simulink model "Model_3_Hieu_1_12"  (R2021a)
settings: Solver=VariableStepAuto  StartTime=0.0  StopTime=10  RelTol=1e-3
InitFcn:
  | ml=0.2;
  | mc=0.5;
  | mt=0.5;
  | g=9.81;
  | l_ref=0.5;
  | l_ini=0.5;
  | l=l_ini;
  | n1=5;n2=1;
  | x_ref=10;
  | 
  | %ADRC' s parameter caculation
  | %b0 = (ml+mc)/(mc*ml +mc*mt+ml*mt); %Hieu
  | b0=(ml+mc)/(mt*mc+2*ml*mc+mt*ml+ml^2+mc^2); %Enhanced-coupling
  | k_ESO = 50;
  | T_set  = 6;
  | 
  | s_cl = -5.85/T_set;
  | Kp   = s_cl^2;
  | Kd   = -2*s_cl;
  | 
  | s_ESO = k_ESO*s_cl;
  | l1        = -3*s_ESO;
  | l2        = 3*( s_ESO)^2;
  | l3        = -(s_ESO)^3;
  | 
  | %Observer
  | A = [-l1, 1, 0;
  |         -l2, 0, 1;
  |         -l3, 0, 0];
  | B = [0;
  |         b0;
  |         0];
  | L = [l1;
  |        l2;
  |        l3];
  | 
  | %b1 = (mt+mc)/(mc*ml +mc*mt+ml*mt);
  | b1=1/(ml+mc);
  | k_ESO1 =100;
  | T_set1  = 3;
  | s_cl1 = -5.85/T_set1;
  | Kp1   = s_cl1^2;
  | Kd1   = -2*s_cl1;
  | 
  | s_ESO1 = k_ESO1*s_cl1;
  | l11        = -3*s_ESO1;
  | l21        = 3*( s_ESO1)^2;
  | l31        = -(s_ESO1)^3;
  | 
  | %Observer
  | A1 = [-l11, 1, 0;
  |         -l21, 0, 1;
  |         -l31, 0, 0];
  | B1 = [0;
  |         b1;
  |         0];
  | L1 = [l11;
  |        l21;
  |        l31];
  | 
  | L1=l_ini;
  | L2=0.2;
  | m1=0.2;
  | m2=0.5;
  | m=0.5;
  | %Bo input shaping
  | alpha = (1/L1 + 1/L2)*(m1+m2)/m1;
  | beta = (((m1+m2)/m1)^2)*((1/L1 + 1/L2)^2) - 4*(m1+m2)/(m1*L1*L2);
  | w1 = sqrt(g*(alpha - sqrt(beta))/2);
  | w2 = sqrt(g*(alpha + sqrt(beta))/2);
  | damping_ratio = 0;
  | wd1 = w1*sqrt(1-damping_ratio^2);
  | wd2 = w2*sqrt(1-damping_ratio^2);
  | k = exp(damping_ratio*pi/sqrt(1-damping_ratio^2));
  | 
  | %ETM4_1
  | m_etm4_1 = 0.1;
  | I_etm4_1 = (1+m_etm4_1)*k*k/(k^2 + (1+m_etm4_1)*(k^(4/3)+k^(2/3)) + m_etm4_1);
  | A1_etm4_1 = I_etm4_1/(1+m_etm4_1);
  | A2_etm4_1 = I_etm4_1/(k^(2/3));
  | A3_etm4_1 = I_etm4_1/(k^(4/3));
  | A4_etm4_1 = m_etm4_1*I_etm4_1/((1+m_etm4_1)*(k^2));
  | t1_etm4_1 = (2*pi/3)/wd1;
  | t2_etm4_1 = (4*pi/3)/wd1;
  | t3_etm4_1 = 2*pi/wd1;
  | %ETM4_2
  | m_etm4_2 = 0.1;
  | I_etm4_2 = (1+m_etm4_2)*k*k/(k^2 + (1+m_etm4_2)*(k^(4/3)+k^(2/3)) + m_etm4_2);
  | A1_etm4_2 = I_etm4_2/(1+m_etm4_2);
  | A2_etm4_2 = I_etm4_2/(k^(2/3));
  | A3_etm4_2 = I_etm4_2/(k^(4/3));
  | A4_etm4_2 = m_etm4_2*I_etm4_2/((1+m_etm4_2)*(k^2));
  | t1_etm4_2 = (2*pi/3)/wd2;
  | t2_etm4_2 = (4*pi/3)/wd2;
  | t3_etm4_2 = 2*pi/wd2;
values from neighbouring files (symbols this model uses):
  particle = repmat(empty_particle, nPop, 1)    [PSO16_12.m]    (also in PSO_ZVD.m)
undefined symbols (not defined in the file or in its folder): i
libraries: neural x35, simulink_extras x11, simulink x5
(part 1 of 15)
settings Model: Creator=Dao Hieu  LastModifiedBy=Admin

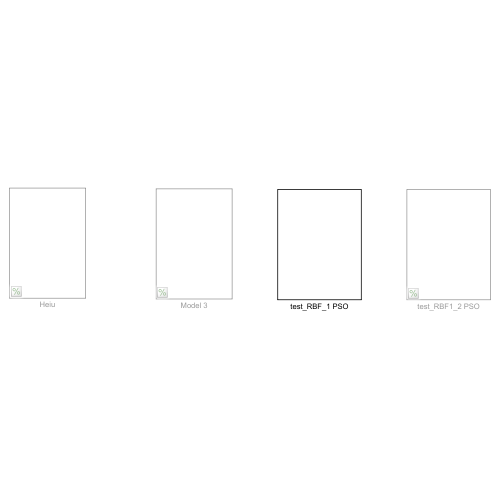
[thumbnail: Simulink's stored preview of the top-level diagram]
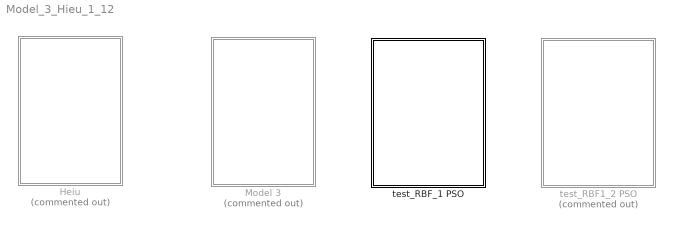
== system Model_3_Hieu_1_12 ==
  Heiu : Subsystem  Commented=on
  Model 3 : Subsystem  Commented=on
  test_RBF1_2 PSO : Subsystem  Commented=on
  test_RBF_1 PSO : Subsystem

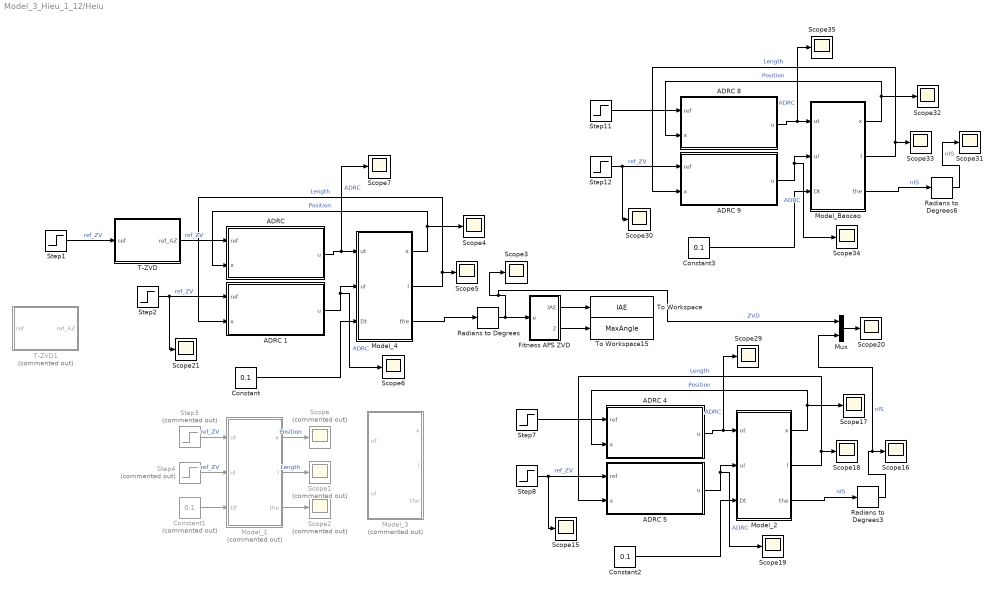
== system Model_3_Hieu_1_12/Heiu ==
  "ADRC " : Subsystem
  ADRC 1 : Subsystem
  ADRC 4 : Subsystem
  ADRC 5 : Subsystem
  ADRC 8 : Subsystem
  ADRC 9 : Subsystem
  Constant : Constant  Value=0.1
  Constant1 : Constant  Commented=on  Value=0.1
  Constant2 : Constant  Value=0.1
  Constant3 : Constant  Value=0.1
  Fitness APS ZVD : Subsystem
  Model_1 : Subsystem  Commented=on
  Model_2 : Subsystem
  Model_3 : Subsystem  Commented=on
  Model_4 : Subsystem
  Model_Baocao : Subsystem
  Mux : Mux  Inputs=2
  Radians to Degrees : simulink_extras/Transformations/Radians to Degrees
  Radians to Degrees3 : simulink_extras/Transformations/Radians to Degrees
  Radians to Degrees6 : simulink_extras/Transformations/Radians to Degrees
  Scope : Scope  Commented=on
  Scope1 : Scope  Commented=on
  Scope{3..7,15..21,29..35} (19 alike) : Scope
  Scope2 : Scope  Commented=on
  Step1 : Step  SampleTime=0
  Step11 : Step  SampleTime=0
  Step12 : Step  Before=l_ini  After=l_ref  SampleTime=0
  Step2 : Step  Before=l_ini  After=l_ref  SampleTime=0
  Step3 : Step  Commented=on  SampleTime=0
  Step4 : Step  Commented=on  Before=l  After=l  SampleTime=0
  Step7 : Step  SampleTime=0
  Step8 : Step  Before=l_ini  After=l_ref  SampleTime=0
  T-ZVD : Subsystem
  T-ZVD1 : Subsystem  Commented=on
  To Workspace : ToWorkspace  VariableName=IAE  SampleTime=-1
  To Workspace15 : ToWorkspace  VariableName=MaxAngle  SampleTime=-1
  wires:
  Model_4/1(x) -> Scope4/1, "ADRC "/2(x)  "Position"
  Model_4/3(the) -> Radians to Degrees/1
  Step12/1 -> Scope30/1, ADRC 9/1(ref)  "ref_ZV"
  "ADRC "/1(u) -> Scope7/1, Model_4/1(ut)  "ADRC"
  Model_Baocao/2(l) -> Scope33/1, ADRC 9/2(x)  "Length"
  Mux/1 -> Scope20/1
  Radians to Degrees6/1 -> Scope31/1  "nIS"
  Model_2/1(x) -> ADRC 4/2(x), Scope17/1  "Position"
  Fitness APS ZVD/1(IAE) -> To Workspace/1
  Step8/1 -> ADRC 5/1(ref), Scope15/1  "ref_ZV"
  Fitness APS ZVD/2(MAx) -> To Workspace15/1
  ADRC 1/1(u) -> Scope6/1, Model_4/2(ul)  "ADRC"
  Step11/1 -> ADRC 8/1(ref)
  Radians to Degrees/1 -> Mux/1, Scope3/1, Fitness APS ZVD/1(e)  "ZVD"
  Constant3/1 -> Model_Baocao/3(Dt)
  Step4/1 -> Model_1/2(ul)  "ref_ZV"
  Step2/1 -> Scope21/1, ADRC 1/1(ref)  "ref_ZV"
  Model_1/1(x) -> Scope/1  "Position"
  ADRC 5/1(u) -> Scope19/1, Model_2/2(ul)  "ADRC"
  Model_2/3(the) -> Radians to Degrees3/1  "nIS"
  Model_1/3(the) -> Scope2/1
  ADRC 8/1(u) -> Scope35/1, Model_Baocao/1(ut)  "ADRC"
  Constant/1 -> Model_4/3(Dt)
  Step1/1 -> T-ZVD/1(ref)  "ref_ZV"
  Step3/1 -> Model_1/1(ut)  "ref_ZV"
  ADRC 4/1(u) -> Scope29/1, Model_2/1(ut)  "ADRC"
  Radians to Degrees3/1 -> Mux/2, Scope16/1  "nIS"
  T-ZVD/1(ref_AZ) -> "ADRC "/1(ref)  "ref_ZV"
  Model_2/2(l) -> ADRC 5/2(x), Scope18/1  "Length"
  ADRC 9/1(u) -> Scope34/1, Model_Baocao/2(ul)  "ADRC"
  Constant2/1 -> Model_2/3(Dt)
  Model_Baocao/1(x) -> Scope32/1, ADRC 8/2(x)  "Position"
  Model_Baocao/3(the) -> Radians to Degrees6/1  "nIS"
  Constant1/1 -> Model_1/3(Dt)
  Step7/1 -> ADRC 4/1(ref)
  Model_1/2(l) -> Scope1/1  "Length"
  Model_4/2(l) -> Scope5/1, ADRC 1/2(x)  "Length"

== system Model_3_Hieu_1_12/Model 3 ==
  ADRC 10 : Subsystem
  ADRC 11 : Subsystem
  ADRC 6 : Subsystem
  ADRC 7 : Subsystem
  ETM2 : Subsystem
  Mux1 : Mux  Inputs=2
  Mux2 : Mux  Inputs=2
  Radians to Degrees{4..5,7..8} (4 alike) : simulink_extras/Transformations/Radians to Degrees
  Scope{22..28,36..43} (15 alike) : Scope
  Step10 : Step  Before=l_ini  After=l_ref  SampleTime=0
  Step13 : Step  Before=l_ini  After=l_ref  SampleTime=0
  Step14 : Step  SampleTime=0
  Step9 : Step  SampleTime=0
  Theta1 : Scope
  Theta2 : Scope
  enhanced : Subsystem
  enhanced1 : Subsystem
  wires:
  Radians to Degrees4/1 -> Mux1/1, Scope28/1  "ET4"
  enhanced1/1(x) -> Scope22/1, ADRC 6/2(x)  "Position"
  enhanced1/3(the1) -> Radians to Degrees4/1
  ADRC 6/1(u) -> Scope25/1, enhanced1/1(Fx)  "ADRC"
  Radians to Degrees7/1 -> Mux1/2, Scope42/1  "nIS"
  Step13/1 -> Scope41/1, ADRC 11/1(ref)  "ref_ZV"
  enhanced/2(l) -> Scope37/1, ADRC 11/2(x)  "Length"
  Radians to Degrees5/1 -> Mux2/1, Scope26/1  "ET4"
  ADRC 11/1(u) -> enhanced/2(Fl), Scope38/1  "ADRC"
  ADRC 7/1(u) -> Scope24/1, enhanced1/2(Fl)  "ADRC"
  ETM2/1(ref_ETM4) -> Scope43/1, ADRC 6/1(ref)  "ref_ZV"
  enhanced/1(x) -> Scope36/1, ADRC 10/2(x)  "Position"
  Step9/1 -> ETM2/1(ref_ETm4)  "ref_ZV"
  Mux1/1 -> Theta1/1
  enhanced1/2(l) -> Scope23/1, ADRC 7/2(x)  "Length"
  Step14/1 -> ADRC 10/1(ref)  "ref_ZV"
  Mux2/1 -> Theta2/1
  enhanced1/4(the2) -> Radians to Degrees5/1
  enhanced/3(the1) -> Radians to Degrees7/1
  Step10/1 -> Scope27/1, ADRC 7/1(ref)  "ref_ZV"
  ADRC 10/1(u) -> enhanced/1(Fx), Scope39/1  "ADRC"
  Radians to Degrees8/1 -> Mux2/2, Scope40/1  "nIS"
  enhanced/4(the2) -> Radians to Degrees8/1

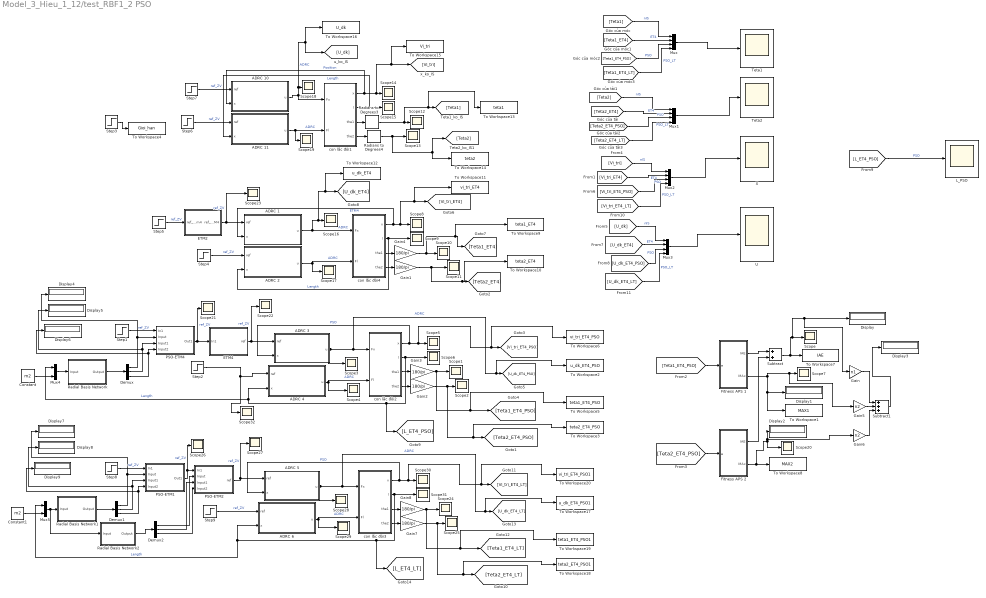
== system Model_3_Hieu_1_12/test_RBF1_2 PSO ==
  ADRC 1 : Subsystem
  ADRC 10 : Subsystem
  ADRC 11 : Subsystem
  ADRC 2 : Subsystem
  ADRC 3 : Subsystem
  ADRC 4 : Subsystem
  ADRC 5 : Subsystem
  ADRC 6 : Subsystem
  Constant : Constant  Value=m2
  Constant1 : Constant  Value=m2
  Demux : Demux  Outputs=3
  Demux1 : Demux  Outputs=3
  Demux2 : Demux  Outputs=3
  Display{,1..9} (10 alike) : Display
  ETM2 : Subsystem
  ETM4 : Subsystem
  Fitness APS 1 : Subsystem
  Fitness APS 2 : Subsystem
  Gain : Gain  Gain=n1
  Gain{1..4,7..8} (6 alike) : Gain  Gain=180/pi
  Gain5 : Gain  Gain=n2
  Gain6 : Gain  Gain=n2
  L_PSO : Scope
  Mux{,1..3} (4 alike) : Mux
  Mux4 : Mux  Inputs=2
  Mux5 : Mux  Inputs=2
  PSO-ETM1 : Subsystem
  PSO-ETM2 : Subsystem
  PSO-ETM4 : Subsystem
  Radial Basis Network : Subsystem
      mask help: Radial Basis Network
      mask Display: e = 0.06;c1 = [120 150 230]/255;c2 = ([120 150 230]+0)/383;c3 = ([120 150 230]+128)/383;patch([0 1 1 0],[0 0 1 1],c1);patch([0 1 1 1-e 1-e 0+e],[0 0 1 1-e 0+e 0+e],c2);patch([0 0 1 1-e 0+e 0+e],[0 1 1 1-e 1-e 0+e],c3);plot([0 1 1 0 0],[0 0 1 1 0]);fprintf('NNET');port_label('input',1,' Input');port_label('output',1,'Output ');
  Radial Basis Network1 : Subsystem
      mask help: Radial Basis Network
      mask Display: e = 0.06;c1 = [120 150 230]/255;c2 = ([120 150 230]+0)/383;c3 = ([120 150 230]+128)/383;patch([0 1 1 0],[0 0 1 1],c1);patch([0 1 1 1-e 1-e 0+e],[0 0 1 1-e 0+e 0+e],c2);patch([0 0 1 1-e 0+e 0+e],[0 1 1 1-e 1-e 0+e],c3);plot([0 1 1 0 0],[0 0 1 1 0]);fprintf('NNET');port_label('input',1,' Input');port_label('output',1,'Output ');
  Radial Basis Network2 : Subsystem
      mask help: Radial Basis Network
      mask Display: e = 0.06;c1 = [120 150 230]/255;c2 = ([120 150 230]+0)/383;c3 = ([120 150 230]+128)/383;patch([0 1 1 0],[0 0 1 1],c1);patch([0 1 1 1-e 1-e 0+e],[0 0 1 1-e 0+e 0+e],c2);patch([0 0 1 1-e 0+e 0+e],[0 1 1 1-e 1-e 0+e],c3);plot([0 1 1 0 0],[0 0 1 1 0]);fprintf('NNET');port_label('input',1,' Input');port_label('output',1,'Output ');
  Radians to Degrees3 : simulink_extras/Transformations/Radians to Degrees
  Radians to Degrees4 : simulink_extras/Transformations/Radians to Degrees
  Scope{,1..32} (33 alike) : Scope
  Step{1,5,7..8} (4 alike) : Step  Time=0  After=x_ref  SampleTime=0
  Step{2,4,6,9} (4 alike) : Step  Time=0  Before=l_ini  After=l_ref  SampleTime=0
  Step3 : Step  Time=0  After=10  SampleTime=0
  Subtract : Sum
  Subtract1 : Sum  Inputs=+++
  Teta1 : Scope
  Teta2 : Scope
  To Workspace1 : ToWorkspace  VariableName=MAX1  SaveFormat=Timeseries  SampleTime=-1
  To Workspace10 : ToWorkspace  VariableName=teta2_ET4  SaveFormat=Timeseries  SampleTime=-1
  To Workspace11 : ToWorkspace  VariableName=vi_tri_ET4  SaveFormat=Timeseries  SampleTime=-1
  To Workspace12 : ToWorkspace  VariableName=u_dk_ET4  SaveFormat=Timeseries  SampleTime=-1
  To Workspace13 : ToWorkspace  VariableName=teta1  SaveFormat=Timeseries  SampleTime=-1
  To Workspace14 : ToWorkspace  VariableName=teta2  SaveFormat=Timeseries  SampleTime=-1
  To Workspace15 : ToWorkspace  VariableName=Vi_tri  SaveFormat=Timeseries  SampleTime=-1
  To Workspace16 : ToWorkspace  VariableName=U_dk  SaveFormat=Timeseries  SampleTime=-1
  To Workspace17 : ToWorkspace  VariableName=u_dk_ET4_PSO1  SaveFormat=Timeseries  SampleTime=-1
  To Workspace18 : ToWorkspace  VariableName=teta2_ET4_PSO1  SaveFormat=Timeseries  SampleTime=-1
  To Workspace19 : ToWorkspace  VariableName=teta1_ET4_PSO1  SaveFormat=Timeseries  SampleTime=-1
  To Workspace2 : ToWorkspace  VariableName=u_dk_ET4_PSO  SaveFormat=Timeseries  SampleTime=-1
  To Workspace20 : ToWorkspace  VariableName=vi_tri_ET4_PSO1  SaveFormat=Timeseries  SampleTime=-1
  To Workspace3 : ToWorkspace  VariableName=teta2_ET4_PSO  SaveFormat=Timeseries  SampleTime=-1
  To Workspace4 : ToWorkspace  VariableName=Gioi_han  SaveFormat=Timeseries  SampleTime=-1
  To Workspace5 : ToWorkspace  VariableName=teta1_ET4_PSO  SaveFormat=Timeseries  SampleTime=-1
  To Workspace6 : ToWorkspace  VariableName=vi_tri_ET4_PSO  SaveFormat=Timeseries  SampleTime=-1
  To Workspace7 : ToWorkspace  VariableName=IAE  SaveFormat=Timeseries  SampleTime=-1
  To Workspace8 : ToWorkspace  VariableName=MAX2  SaveFormat=Timeseries  SampleTime=-1
  To Workspace9 : ToWorkspace  VariableName=teta1_ET4  SaveFormat=Timeseries  SampleTime=-1
  U : Scope
  X : Scope
  con lắc đôi1 : Subsystem
  con lắc đôi2 : Subsystem
  con lắc đôi3 : Subsystem
  con lắc đôi4 : Subsystem
  wires:
  ADRC 2/1(u) -> con lắc đôi4/2(Fl), Scope17/1  "ADRC"
  ADRC 11/1(u) -> con lắc đôi1/2(Fl), Scope19/1  "ADRC"
  ADRC 1/1(u) -> con lắc đôi4/1(Fx), To Workspace12/1, [U_dk_ET4], Scope16/1  "ADRC"
  con lắc đôi4/1(x) -> ADRC 1/2(x), To Workspace11/1, [Vi_tri_ET4], Scope8/1  "ETM4"
  con lắc đôi1/3(the1) -> Radians to Degrees3/1
  con lắc đôi4/2(l) -> ADRC 2/2(x), Scope9/1  "Length"
  con lắc đôi1/1(x) -> ADRC 10/2(x), To Workspace15/1, [Vi_tri], Scope14/1  "Position"
  Step6/1 -> ADRC 11/1(ref)  "ref_ZV"
  Step4/1 -> ADRC 2/1(ref)  "ref_ZV"
  con lắc đôi1/2(l) -> ADRC 11/2(x), Scope15/1  "Length"
  Step7/1 -> ADRC 10/1(ref)  "ref_ZV"
  Gain4/1 -> To Workspace9/1, [Teta1_ET4], Scope10/1
  ETM2/1(ref_ETM4) -> ADRC 1/1(ref), Scope23/1  "ref_ZV"
  Step5/1 -> ETM2/1(ref_ETm4)  "ref_ZV"
  ADRC 10/1(u) -> con lắc đôi1/1(Fx), To Workspace16/1, [U_dk], Scope18/1  "ADRC"
  Radians to Degrees3/1 -> To Workspace13/1, [Teta1], Scope12/1
  con lắc đôi1/4(the2) -> Radians to Degrees4/1
  con lắc đôi4/3(the1) -> Gain4/1
  Gain1/1 -> To Workspace10/1, [Teta2_ET4], Scope11/1
  con lắc đôi4/4(the2) -> Gain1/1
  Radians to Degrees4/1 -> [Teta2], To Workspace14/1, Scope13/1
  ADRC 4/1(u) -> Scope4/1, con lắc đôi2/2(Fl)  "ADRC"
  con lắc đôi2/4(the2) -> Gain2/1
  Step1/1 -> PSO-ETM4/1(In1)  "ref_ZV"
  ADRC 3/1(u) -> Scope3/1, To Workspace2/1, [U_dk_ET4_PSO], con lắc đôi2/1(Fx)  "ADRC"
  con lắc đôi2/1(x) -> ADRC 3/2(x), To Workspace6/1, [Vi_tri_ET4_PSO], Scope5/1  "PSO"
  con lắc đôi2/2(l) -> Scope6/1, [L_ET4_PSO], ADRC 4/2(x), Mux4/1  "Length"
  Gain3/1 -> [Teta1_ET4_PSO], To Workspace5/1, Scope1/1
  con lắc đôi2/3(the1) -> Gain3/1
  PSO-ETM4/1(Out1) -> Scope21/1, ETM4/1(In1)  "ref_ZV"
  [Teta2] -> Mux1/1  "nIS"
  Subtract/1 -> To Workspace7/1, Gain/1, Display/1, Scope/1
  [U_dk] -> Mux3/1  "nIS"
  [U_dk_ET4] -> Mux3/2  "ET4"
  [Teta2_ET4_PSO] -> Fitness APS 2/1(e)
  [Teta1_ET4_PSO] -> Fitness APS 1/1(e)
  [Vi_tri] -> Mux2/1  "nIS"
  [Teta2_ET4] -> Mux1/2  "ET4"
  [Vi_tri_ET4] -> Mux2/2  "ET4"
  [Teta1] -> Mux/1  "nIS"
  Gain5/1 -> Subtract1/2
  Fitness APS 2/2(MAx) -> To Workspace8/1, Gain6/1, Display2/1, Scope20/1
  Mux2/1 -> X/1
  Gain6/1 -> Subtract1/3
  Mux/1 -> Teta1/1
  Mux1/1 -> Teta2/1
  Mux3/1 -> U/1
  Gain/1 -> Subtract1/1
  [Teta1_ET4] -> Mux/2  "ET4"
  Fitness APS 2/1(IAE) -> Subtract/2
  Subtract1/1 -> Display3/1
  Fitness APS 1/1(IAE) -> Subtract/1
  Fitness APS 1/2(MAx) -> To Workspace1/1, Display1/1, Gain5/1, Scope7/1
  Step3/1 -> To Workspace4/1
  Gain2/1 -> [Teta2_ET4_PSO], To Workspace3/1, Scope2/1
  [Teta2_ET4_PSO] -> Mux1/3  "PSO"
  [Vi_tri_ET4_PSO] -> Mux2/3  "PSO"
  [Teta1_ET4_PSO] -> Mux/3  "PSO"
  [U_dk_ET4_PSO] -> Mux3/3  "PSO"
  Constant/1 -> Mux4/2
  Mux4/1 -> Radial Basis Network/1(Input)
  Demux/1 -> PSO-ETM4/2(Input), Display4/1
  Demux/2 -> Display5/1, PSO-ETM4/3(Input1)
  Demux/3 -> Display6/1, PSO-ETM4/4(Input2)
  [L_ET4_PSO] -> L_PSO/1  "PSO"
  ETM4/1(ref) -> ADRC 3/1(ref), Scope22/1  "ref_ZV"
  Radial Basis Network/1(Output) -> Demux/1
  Demux1/1 -> PSO-ETM1/2(Input), Display7/1
  Mux5/1 -> Radial Basis Network2/1(Input), Radial Basis Network1/1(Input)
  Constant1/1 -> Mux5/2
  con lắc đôi3/1(x) -> ADRC 5/2(x), To Workspace20/1, [Vi_tri_ET4_LT], Scope30/1  "PSO"
  Gain7/1 -> [Teta2_ET4_LT], To Workspace18/1, Scope25/1
  con lắc đôi3/3(the1) -> Gain8/1
  Step9/1 -> ADRC 6/1(ref)  "ref_ZV"
  PSO-ETM2/1(ref) -> ADRC 5/1(ref), Scope27/1  "ref_ZV"
  PSO-ETM1/1(Out1) -> PSO-ETM2/1(In1), Scope26/1  "ref_ZV"
  ADRC 5/1(u) -> Scope28/1, con lắc đôi3/1(Fx), To Workspace17/1, [U_dk_ET4_LT]  "ADRC"
  Demux1/2 -> Display8/1, PSO-ETM1/3(Input1)
  Demux1/3 -> Display9/1, PSO-ETM1/4(Input2)
  ADRC 6/1(u) -> con lắc đôi3/2(Fl), Scope29/1  "ADRC"
  con lắc đôi3/2(l) -> Scope31/1, [L_ET4_LT], ADRC 6/2(x), Mux5/1  "Length"
  Radial Basis Network1/1(Output) -> Demux1/1
  Gain8/1 -> [Teta1_ET4_LT], To Workspace19/1, Scope24/1
  con lắc đôi3/4(the2) -> Gain7/1
  Step8/1 -> PSO-ETM1/1(In1)  "ref_ZV"
  [Teta1_ET4_LT] -> Mux/4  "PSO_LT"
  [Teta2_ET4_LT] -> Mux1/4  "PSO_LT"
  [Vi_tri_ET4_LT] -> Mux2/4  "PSO_LT"
  [U_dk_ET4_LT] -> Mux3/4  "PSO_LT"
  Radial Basis Network2/1(Output) -> Demux2/1
  Demux2/1 -> PSO-ETM2/2(Input)
  Demux2/2 -> PSO-ETM2/3(Input1)
  Demux2/3 -> PSO-ETM2/4(Input2)
  Step2/1 -> Scope32/1, ADRC 4/1(ref)

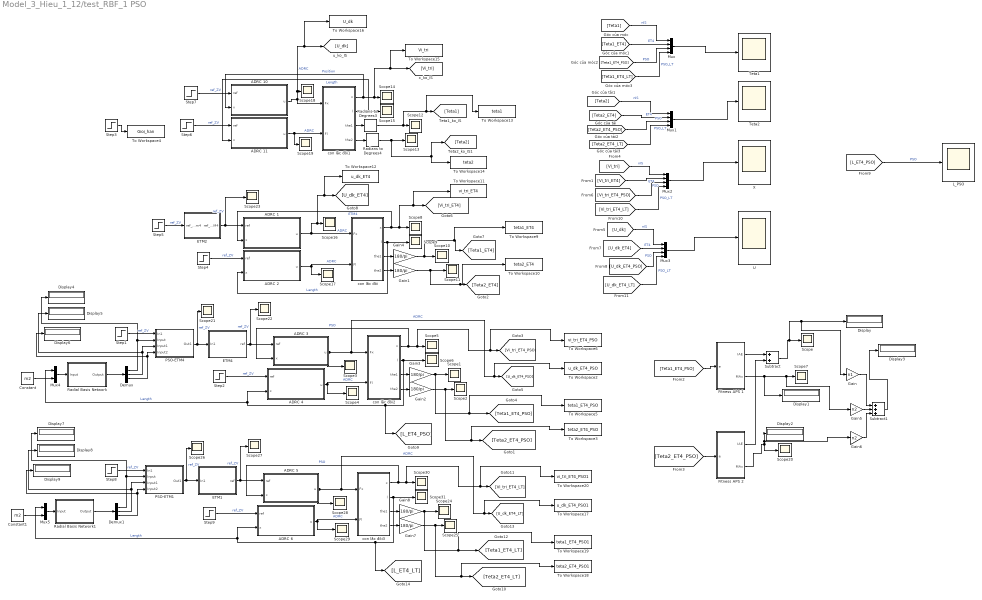
== system Model_3_Hieu_1_12/test_RBF_1 PSO ==
  ADRC 1 : Subsystem
  ADRC 10 : Subsystem
  ADRC 11 : Subsystem
  ADRC 2 : Subsystem
  ADRC 3 : Subsystem
  ADRC 4 : Subsystem
  ADRC 5 : Subsystem
  ADRC 6 : Subsystem
  Constant : Constant  Value=m2
  Constant1 : Constant  Value=m2
  Demux : Demux  Outputs=3
  Demux1 : Demux  Outputs=3
  Display{,1..9} (10 alike) : Display
  ETM1 : Subsystem
  ETM2 : Subsystem
  ETM4 : Subsystem
  Fitness APS 1 : Subsystem
  Fitness APS 2 : Subsystem
  Gain : Gain  Gain=n1
  Gain{1..4,7..8} (6 alike) : Gain  Gain=180/pi
  Gain5 : Gain  Gain=n2
  Gain6 : Gain  Gain=n2
  L_PSO : Scope
  Mux{,1..3} (4 alike) : Mux
  Mux4 : Mux  Inputs=2
  Mux5 : Mux  Inputs=2
  PSO-ETM1 : Subsystem
  PSO-ETM4 : Subsystem
  Radial Basis Network : Subsystem
      mask help: Radial Basis Network
      mask Display: e = 0.06;c1 = [120 150 230]/255;c2 = ([120 150 230]+0)/383;c3 = ([120 150 230]+128)/383;patch([0 1 1 0],[0 0 1 1],c1);patch([0 1 1 1-e 1-e 0+e],[0 0 1 1-e 0+e 0+e],c2);patch([0 0 1 1-e 0+e 0+e],[0 1 1 1-e 1-e 0+e],c3);plot([0 1 1 0 0],[0 0 1 1 0]);fprintf('NNET');port_label('input',1,' Input');port_label('output',1,'Output ');
  Radial Basis Network1 : Subsystem
      mask help: Radial Basis Network
      mask Display: e = 0.06;c1 = [120 150 230]/255;c2 = ([120 150 230]+0)/383;c3 = ([120 150 230]+128)/383;patch([0 1 1 0],[0 0 1 1],c1);patch([0 1 1 1-e 1-e 0+e],[0 0 1 1-e 0+e 0+e],c2);patch([0 0 1 1-e 0+e 0+e],[0 1 1 1-e 1-e 0+e],c3);plot([0 1 1 0 0],[0 0 1 1 0]);fprintf('NNET');port_label('input',1,' Input');port_label('output',1,'Output ');
  Radians to Degrees3 : simulink_extras/Transformations/Radians to Degrees
  Radians to Degrees4 : simulink_extras/Transformations/Radians to Degrees
  Scope{,1..31} (32 alike) : Scope
  Step{1,5,7..8} (4 alike) : Step  Time=0  After=x_ref  SampleTime=0
  Step{2,4,6,9} (4 alike) : Step  Time=0  Before=l_ini  After=l_ref  SampleTime=0
  Step3 : Step  Time=0  After=10  SampleTime=0
  Subtract : Sum
  Subtract1 : Sum  Inputs=+++
  Teta1 : Scope
  Teta2 : Scope
  To Workspace10 : ToWorkspace  VariableName=teta2_ET4  SaveFormat=Timeseries  SampleTime=-1
  To Workspace11 : ToWorkspace  VariableName=vi_tri_ET4  SaveFormat=Timeseries  SampleTime=-1
  To Workspace12 : ToWorkspace  VariableName=u_dk_ET4  SaveFormat=Timeseries  SampleTime=-1
  To Workspace13 : ToWorkspace  VariableName=teta1  SaveFormat=Timeseries  SampleTime=-1
  To Workspace14 : ToWorkspace  VariableName=teta2  SaveFormat=Timeseries  SampleTime=-1
  To Workspace15 : ToWorkspace  VariableName=Vi_tri  SaveFormat=Timeseries  SampleTime=-1
  To Workspace16 : ToWorkspace  VariableName=U_dk  SaveFormat=Timeseries  SampleTime=-1
  To Workspace17 : ToWorkspace  VariableName=u_dk_ET4_PSO1  SaveFormat=Timeseries  SampleTime=-1
  To Workspace18 : ToWorkspace  VariableName=teta2_ET4_PSO1  SaveFormat=Timeseries  SampleTime=-1
  To Workspace19 : ToWorkspace  VariableName=teta1_ET4_PSO1  SaveFormat=Timeseries  SampleTime=-1
  To Workspace2 : ToWorkspace  VariableName=u_dk_ET4_PSO  SaveFormat=Timeseries  SampleTime=-1
  To Workspace20 : ToWorkspace  VariableName=vi_tri_ET4_PSO1  SaveFormat=Timeseries  SampleTime=-1
  To Workspace3 : ToWorkspace  VariableName=teta2_ET4_PSO  SaveFormat=Timeseries  SampleTime=-1
  To Workspace4 : ToWorkspace  VariableName=Gioi_han  SaveFormat=Timeseries  SampleTime=-1
  To Workspace5 : ToWorkspace  VariableName=teta1_ET4_PSO  SaveFormat=Timeseries  SampleTime=-1
  To Workspace6 : ToWorkspace  VariableName=vi_tri_ET4_PSO  SaveFormat=Timeseries  SampleTime=-1
  To Workspace9 : ToWorkspace  VariableName=teta1_ET4  SaveFormat=Timeseries  SampleTime=-1
  U : Scope
  X : Scope
  con lắc đôi : Subsystem
  con lắc đôi1 : Subsystem
  con lắc đôi2 : Subsystem
  con lắc đôi3 : Subsystem
  wires:
  ADRC 2/1(u) -> Scope17/1, con lắc đôi/2(Fl)  "ADRC"
  ADRC 11/1(u) -> con lắc đôi1/2(Fl), Scope19/1  "ADRC"
  ADRC 1/1(u) -> To Workspace12/1, [U_dk_ET4], Scope16/1, con lắc đôi/1(Fx)  "ADRC"
  con lắc đôi/1(x) -> ADRC 1/2(x), To Workspace11/1, [Vi_tri_ET4], Scope8/1  "ETM4"
  con lắc đôi1/3(the1) -> Radians to Degrees3/1
  con lắc đôi/2(l) -> ADRC 2/2(x), Scope9/1  "Length"
  con lắc đôi1/1(x) -> ADRC 10/2(x), To Workspace15/1, [Vi_tri], Scope14/1  "Position"
  Step6/1 -> ADRC 11/1(ref)  "ref_ZV"
  Step4/1 -> ADRC 2/1(ref)  "ref_ZV"
  con lắc đôi1/2(l) -> ADRC 11/2(x), Scope15/1  "Length"
  Step7/1 -> ADRC 10/1(ref)  "ref_ZV"
  Gain4/1 -> To Workspace9/1, [Teta1_ET4], Scope10/1
  ETM2/1(ref_ETM4) -> ADRC 1/1(ref), Scope23/1  "ref_ZV"
  Step5/1 -> ETM2/1(ref_ETm4)  "ref_ZV"
  ADRC 10/1(u) -> con lắc đôi1/1(Fx), To Workspace16/1, [U_dk], Scope18/1  "ADRC"
  Radians to Degrees3/1 -> To Workspace13/1, [Teta1], Scope12/1
  con lắc đôi1/4(the2) -> Radians to Degrees4/1
  con lắc đôi/3(the1) -> Gain4/1
  Gain1/1 -> To Workspace10/1, [Teta2_ET4], Scope11/1
  con lắc đôi/4(the2) -> Gain1/1
  Radians to Degrees4/1 -> [Teta2], To Workspace14/1, Scope13/1
  ADRC 4/1(u) -> Scope4/1, con lắc đôi2/2(Fl)  "ADRC"
  con lắc đôi2/4(the2) -> Gain2/1
  Step1/1 -> PSO-ETM4/1(In1)  "ref_ZV"
  ADRC 3/1(u) -> Scope3/1, To Workspace2/1, [U_dk_ET4_PSO], con lắc đôi2/1(Fx)  "ADRC"
  con lắc đôi2/1(x) -> ADRC 3/2(x), To Workspace6/1, [Vi_tri_ET4_PSO], Scope5/1  "PSO"
  con lắc đôi2/2(l) -> Scope6/1, [L_ET4_PSO], ADRC 4/2(x), Mux4/1  "Length"
  Gain3/1 -> [Teta1_ET4_PSO], To Workspace5/1, Scope1/1
  Step2/1 -> ADRC 4/1(ref)  "ref_ZV"
  con lắc đôi2/3(the1) -> Gain3/1
  PSO-ETM4/1(Out1) -> Scope21/1, ETM4/1(In1)  "ref_ZV"
  [Teta2] -> Mux1/1  "nIS"
  Subtract/1 -> Gain/1, Display/1, Scope/1
  [U_dk] -> Mux3/1  "nIS"
  [U_dk_ET4] -> Mux3/2  "ET4"
  [Teta2_ET4_PSO] -> Fitness APS 2/1(e)
  [Teta1_ET4_PSO] -> Fitness APS 1/1(e)
  [Vi_tri] -> Mux2/1  "nIS"
  [Teta2_ET4] -> Mux1/2  "ET4"
  [Vi_tri_ET4] -> Mux2/2  "ET4"
  [Teta1] -> Mux/1  "nIS"
  Gain5/1 -> Subtract1/2
  Fitness APS 2/2(MAx) -> Gain6/1, Display2/1, Scope20/1
  Mux2/1 -> X/1
  Gain6/1 -> Subtract1/3
  Mux/1 -> Teta1/1
  Mux1/1 -> Teta2/1
  Mux3/1 -> U/1
  Gain/1 -> Subtract1/1
  [Teta1_ET4] -> Mux/2  "ET4"
  Fitness APS 2/1(IAE) -> Subtract/2
  Subtract1/1 -> Display3/1
  Fitness APS 1/1(IAE) -> Subtract/1
  Fitness APS 1/2(MAx) -> Display1/1, Gain5/1, Scope7/1
  Step3/1 -> To Workspace4/1
  Gain2/1 -> [Teta2_ET4_PSO], To Workspace3/1, Scope2/1
  [Teta2_ET4_PSO] -> Mux1/3  "PSO"
  [Vi_tri_ET4_PSO] -> Mux2/3  "PSO"
  [Teta1_ET4_PSO] -> Mux/3  "PSO"
  [U_dk_ET4_PSO] -> Mux3/3  "PSO"
  Constant/1 -> Mux4/2
  Mux4/1 -> Radial Basis Network/1(Input)
  Demux/1 -> PSO-ETM4/2(Input), Display4/1
  Demux/2 -> Display5/1, PSO-ETM4/3(Input1)
  Demux/3 -> Display6/1, PSO-ETM4/4(Input2)
  [L_ET4_PSO] -> L_PSO/1  "PSO"
  ETM4/1(ref) -> ADRC 3/1(ref), Scope22/1  "ref_ZV"
  Radial Basis Network/1(Output) -> Demux/1
  Demux1/1 -> PSO-ETM1/2(Input), Display7/1
  Mux5/1 -> Radial Basis Network1/1(Input)
  Constant1/1 -> Mux5/2
  con lắc đôi3/1(x) -> ADRC 5/2(x), To Workspace20/1, [Vi_tri_ET4_LT], Scope30/1  "PSO"
  Gain7/1 -> [Teta2_ET4_LT], To Workspace18/1, Scope25/1
  con lắc đôi3/3(the1) -> Gain8/1
  Step9/1 -> ADRC 6/1(ref)  "ref_ZV"
  ETM1/1(ref) -> ADRC 5/1(ref), Scope27/1  "ref_ZV"
  PSO-ETM1/1(Out1) -> Scope26/1, ETM1/1(In1)  "ref_ZV"
  ADRC 5/1(u) -> Scope28/1, To Workspace17/1, [U_dk_ET4_LT], con lắc đôi3/1(Fx)  "ADRC"
  Demux1/2 -> Display8/1, PSO-ETM1/3(Input1)
  Demux1/3 -> Display9/1, PSO-ETM1/4(Input2)
  ADRC 6/1(u) -> Scope29/1, con lắc đôi3/2(Fl)  "ADRC"
  con lắc đôi3/2(l) -> Scope31/1, [L_ET4_LT], ADRC 6/2(x), Mux5/1  "Length"
  Radial Basis Network1/1(Output) -> Demux1/1
  Gain8/1 -> [Teta1_ET4_LT], To Workspace19/1, Scope24/1
  con lắc đôi3/4(the2) -> Gain7/1
  Step8/1 -> PSO-ETM1/1(In1)  "ref_ZV"
  [Teta1_ET4_LT] -> Mux/4  "PSO_LT"
  [Teta2_ET4_LT] -> Mux1/4  "PSO_LT"
  [Vi_tri_ET4_LT] -> Mux2/4  "PSO_LT"
  [U_dk_ET4_LT] -> Mux3/4  "PSO_LT"

== system Model_3_Hieu_1_12/Heiu/ADRC  ==
  ref : Inport
  x : Inport  Port=2
  Gain : Gain  Gain=Kp
  Gain1 : Gain  Gain=Kd
  Gain2 : Gain  Gain=1/b0
  Observer : Subsystem
  Sum : Sum  Inputs=|+-
  Sum3 : Sum  Inputs=|+-
  Sum4 : Sum  Inputs=|+-
  u : Outport
  wires:
  Sum4/1 -> Gain2/1
  Sum/1 -> Gain/1
  Gain2/1 -> u/1, Observer/1(u)
  x/1 -> Observer/2(x)
  Sum3/1 -> Sum4/1
  Observer/2(x2) -> Gain1/1
  Gain1/1 -> Sum3/2
  Gain/1 -> Sum3/1
  ref/1 -> Sum/1
  Observer/1(x3) -> Sum4/2
  Observer/3(x1) -> Sum/2

== system Model_3_Hieu_1_12/Heiu/ADRC 1 ==
  ref : Inport
  x : Inport  Port=2
  Gain : Gain  Gain=Kp1
  Gain1 : Gain  Gain=Kd1
  Gain2 : Gain  Gain=1/b1
  Observer : Subsystem
  Sum : Sum  Inputs=|+-
  Sum3 : Sum  Inputs=|+-
  Sum4 : Sum  Inputs=|+-
  u : Outport
  wires:
  Sum4/1 -> Gain2/1
  Sum/1 -> Gain/1
  Gain2/1 -> u/1, Observer/1(u)
  x/1 -> Observer/2(x)
  Sum3/1 -> Sum4/1
  Observer/2(x2) -> Gain1/1
  Gain1/1 -> Sum3/2
  Gain/1 -> Sum3/1
  ref/1 -> Sum/1
  Observer/1(x3) -> Sum4/2
  Observer/3(x1) -> Sum/2

== system Model_3_Hieu_1_12/Heiu/ADRC 4 ==
  ref : Inport
  x : Inport  Port=2
  Gain : Gain  Gain=Kp
  Gain1 : Gain  Gain=Kd
  Gain2 : Gain  Gain=1/b0
  Observer : Subsystem
  Sum : Sum  Inputs=|+-
  Sum3 : Sum  Inputs=|+-
  Sum4 : Sum  Inputs=|+-
  u : Outport
  wires:
  Sum4/1 -> Gain2/1
  Sum/1 -> Gain/1
  Gain2/1 -> u/1, Observer/1(u)
  x/1 -> Observer/2(x)
  Sum3/1 -> Sum4/1
  Observer/2(x2) -> Gain1/1
  Gain1/1 -> Sum3/2
  Gain/1 -> Sum3/1
  ref/1 -> Sum/1
  Observer/1(x3) -> Sum4/2
  Observer/3(x1) -> Sum/2

== system Model_3_Hieu_1_12/Heiu/ADRC 5 ==
  ref : Inport
  x : Inport  Port=2
  Gain : Gain  Gain=Kp1
  Gain1 : Gain  Gain=Kd1
  Gain2 : Gain  Gain=1/b1
  Observer : Subsystem
  Sum : Sum  Inputs=|+-
  Sum3 : Sum  Inputs=|+-
  Sum4 : Sum  Inputs=|+-
  u : Outport
  wires:
  Sum4/1 -> Gain2/1
  Sum/1 -> Gain/1
  Gain2/1 -> u/1, Observer/1(u)
  x/1 -> Observer/2(x)
  Sum3/1 -> Sum4/1
  Observer/2(x2) -> Gain1/1
  Gain1/1 -> Sum3/2
  Gain/1 -> Sum3/1
  ref/1 -> Sum/1
  Observer/1(x3) -> Sum4/2
  Observer/3(x1) -> Sum/2

== system Model_3_Hieu_1_12/Heiu/ADRC 8 ==
  ref : Inport
  x : Inport  Port=2
  Gain : Gain  Gain=Kp
  Gain1 : Gain  Gain=Kd
  Gain2 : Gain  Gain=1/b0
  Observer : Subsystem
  Sum : Sum  Inputs=|+-
  Sum3 : Sum  Inputs=|+-
  Sum4 : Sum  Inputs=|+-
  u : Outport
  wires:
  Sum4/1 -> Gain2/1
  Sum/1 -> Gain/1
  Gain2/1 -> u/1, Observer/1(u)
  x/1 -> Observer/2(x)
  Sum3/1 -> Sum4/1
  Observer/2(x2) -> Gain1/1
  Gain1/1 -> Sum3/2
  Gain/1 -> Sum3/1
  ref/1 -> Sum/1
  Observer/1(x3) -> Sum4/2
  Observer/3(x1) -> Sum/2

== system Model_3_Hieu_1_12/Heiu/ADRC 9 ==
  ref : Inport
  x : Inport  Port=2
  Gain : Gain  Gain=Kp1
  Gain1 : Gain  Gain=Kd1
  Gain2 : Gain  Gain=1/b1
  Observer : Subsystem
  Sum : Sum  Inputs=|+-
  Sum3 : Sum  Inputs=|+-
  Sum4 : Sum  Inputs=|+-
  u : Outport
  wires:
  Sum4/1 -> Gain2/1
  Sum/1 -> Gain/1
  Gain2/1 -> u/1, Observer/1(u)
  x/1 -> Observer/2(x)
  Sum3/1 -> Sum4/1
  Observer/2(x2) -> Gain1/1
  Gain1/1 -> Sum3/2
  Gain/1 -> Sum3/1
  ref/1 -> Sum/1
  Observer/1(x3) -> Sum4/2
  Observer/3(x1) -> Sum/2

== system Model_3_Hieu_1_12/Heiu/Fitness APS ZVD ==
  e : Inport
  Abs : Abs
  Abs1 : Abs
  Integrator : Integrator
  MinMax Running Resettable : simulink/Math Operations/MinMax Running Resettable  Function=max  vinit=0.0
  Step : Step  Time=0.000001  Before=1  After=0  SampleTime=0
  IAE : Outport
  MAx : Outport  Port=2
  wires:
  Abs/1 -> Integrator/1
  Abs1/1 -> MinMax Running Resettable/1
  Step/1 -> MinMax Running Resettable/2
  e/1 -> Abs/1, Abs1/1
  Integrator/1 -> IAE/1
  MinMax Running Resettable/1 -> MAx/1

== system Model_3_Hieu_1_12/Heiu/Model_1 ==
  ut : Inport
  ul : Inport  Port=2
  Dt : Inport  Port=3
  Add : Sum
  Constant : Constant  Value=-mc*g
  Constant1 : Constant  Value=mc
  Crane : MATLAB Function  TreatAsAtomicUnit=on
  Integrator{,1,3..5} (5 alike) : Integrator
  Integrator2 : Integrator  InitialCondition=l
  x : Outport
  l : Outport  Port=2
  the : Outport  Port=3
  wires:
  Integrator5/1 -> [x6]
  Integrator2/1 -> l/1, [x3]
  [x4] -> Crane/3(x4)
  Crane/1(dx1) -> Integrator/1
  Integrator1/1 -> [x2]
  [x2] -> Crane/1(x2)
  Integrator4/1 -> the/1, [x5]
  [x3] -> Crane/2(x3)
  [x6] -> Crane/5(x6)
  [x5] -> Crane/4(x5)
  Integrator/1 -> x/1, [x1]
  Integrator3/1 -> [x4]
  Crane/2(dx2) -> Integrator1/1
  ut/1 -> Crane/6(ut)
  ul/1 -> Add/2
  Constant/1 -> Add/1
  Add/1 -> Crane/7(ul)
  Crane/3(dx3) -> Integrator2/1
  Crane/4(dx4) -> Integrator3/1
  Crane/5(dx5) -> Integrator4/1
  Crane/6(dx6) -> Integrator5/1
  Dt/1 -> Crane/8(Dt)
  Constant1/1 -> Crane/9(mc)

== system Model_3_Hieu_1_12/Heiu/Model_2 ==
  ut : Inport
  ul : Inport  Port=2
  Dt : Inport  Port=3
  Add : Sum
  Constant : Constant  Value=-mc*g
  Constant1 : Constant  Value=mc
  Crane : MATLAB Function  TreatAsAtomicUnit=on
  Integrator{,1,3..5} (5 alike) : Integrator
  Integrator2 : Integrator  InitialCondition=l
  x : Outport
  l : Outport  Port=2
  the : Outport  Port=3
  wires:
  Integrator5/1 -> [x6]
  Integrator2/1 -> l/1, [x3]
  [x4] -> Crane/3(x4)
  Crane/1(dx1) -> Integrator/1
  Integrator1/1 -> [x2]
  [x2] -> Crane/1(x2)
  Integrator4/1 -> the/1, [x5]
  [x3] -> Crane/2(x3)
  [x6] -> Crane/5(x6)
  [x5] -> Crane/4(x5)
  Integrator/1 -> x/1, [x1]
  Integrator3/1 -> [x4]
  Crane/2(dx2) -> Integrator1/1
  ut/1 -> Crane/6(ut)
  ul/1 -> Add/2
  Constant/1 -> Add/1
  Add/1 -> Crane/7(ul)
  Crane/3(dx3) -> Integrator2/1
  Crane/4(dx4) -> Integrator3/1
  Crane/5(dx5) -> Integrator4/1
  Crane/6(dx6) -> Integrator5/1
  Dt/1 -> Crane/8(Dt)
  Constant1/1 -> Crane/9(mc)

== system Model_3_Hieu_1_12/Heiu/Model_3 ==
  ut : Inport
  ul : Inport  Port=2
  Add : Sum
  Constant : Constant  Value=-mc*g
  Crane : MATLAB Function  TreatAsAtomicUnit=on
  Integrator{,1,3..5} (5 alike) : Integrator
  Integrator2 : Integrator  InitialCondition=l
  x : Outport
  l : Outport  Port=2
  the : Outport  Port=3
  wires:
  Integrator5/1 -> [x6]
  Integrator2/1 -> l/1, [x3]
  [x4] -> Crane/4(x4)
  Crane/5(dx5) -> Integrator4/1
  Crane/6(dx6) -> Integrator5/1
  Crane/1(dx1) -> Integrator/1
  Crane/3(dx3) -> Integrator2/1
  Integrator1/1 -> [x2]
  [x2] -> Crane/2(x2)
  Integrator4/1 -> the/1, [x5]
  [x3] -> Crane/3(x3)
  [x6] -> Crane/6(x6)
  [x5] -> Crane/5(x5)
  Crane/4(dx4) -> Integrator3/1
  Integrator/1 -> x/1, [x1]
  Integrator3/1 -> [x4]
  [x1] -> Crane/1(x1)
  Crane/2(dx2) -> Integrator1/1
  ut/1 -> Crane/7(ut)
  ul/1 -> Add/2
  Constant/1 -> Add/1
  Add/1 -> Crane/8(ul)

== system Model_3_Hieu_1_12/Heiu/Model_4 ==
  ut : Inport
  ul : Inport  Port=2
  Dt : Inport  Port=3
  Add : Sum
  Constant : Constant  Value=-mc*g
  Constant1 : Constant  Value=mc
  Crane : MATLAB Function  TreatAsAtomicUnit=on
  Integrator{,1,3..5} (5 alike) : Integrator
  Integrator2 : Integrator  InitialCondition=l
  x : Outport
  l : Outport  Port=2
  the : Outport  Port=3
  wires:
  Integrator5/1 -> [x6]
  Integrator2/1 -> l/1, [x3]
  [x4] -> Crane/3(x4)
  Crane/1(dx1) -> Integrator/1
  Integrator1/1 -> [x2]
  [x2] -> Crane/1(x2)
  Integrator4/1 -> the/1, [x5]
  [x3] -> Crane/2(x3)
  [x6] -> Crane/5(x6)
  [x5] -> Crane/4(x5)
  Integrator/1 -> x/1, [x1]
  Integrator3/1 -> [x4]
  Crane/2(dx2) -> Integrator1/1
  ut/1 -> Crane/6(ut)
  ul/1 -> Add/2
  Constant/1 -> Add/1
  Add/1 -> Crane/7(ul)
  Crane/3(dx3) -> Integrator2/1
  Crane/4(dx4) -> Integrator3/1
  Crane/5(dx5) -> Integrator4/1
  Crane/6(dx6) -> Integrator5/1
  Dt/1 -> Crane/8(Dt)
  Constant1/1 -> Crane/9(mc)

== system Model_3_Hieu_1_12/Heiu/Model_Baocao ==
  ut : Inport
  ul : Inport  Port=2
  Dt : Inport  Port=3
  Add : Sum
  Constant : Constant  Value=-mc*g
  Constant1 : Constant  Value=mc
  Crane : MATLAB Function  TreatAsAtomicUnit=on
  Integrator{,1,3..5} (5 alike) : Integrator
  Integrator2 : Integrator  InitialCondition=l
  x : Outport
  l : Outport  Port=2
  the : Outport  Port=3
  wires:
  Integrator5/1 -> [x6]
  Integrator2/1 -> l/1, [x3]
  Crane/1(dx1) -> Integrator/1
  Integrator1/1 -> [x2]
  Integrator4/1 -> the/1, [x5]
  Integrator/1 -> x/1
  Integrator3/1 -> [x4]
  Crane/2(dx2) -> Integrator1/1
  ut/1 -> Crane/6(Fx)
  ul/1 -> Add/2
  Constant/1 -> Add/1
  Add/1 -> Crane/7(Fl)
  Crane/3(dx3) -> Integrator2/1
  Crane/4(dx4) -> Integrator3/1
  Crane/5(dx5) -> Integrator4/1
  Crane/6(dx6) -> Integrator5/1
  Dt/1 -> Crane/8(bc)
  Constant1/1 -> Crane/9(mp)
  [x2] -> Crane/1(d1x)
  [x3] -> Crane/2(l)
  [x4] -> Crane/3(d1l)
  [x5] -> Crane/4(the)
  [x6] -> Crane/5(d1the)

== system Model_3_Hieu_1_12/Heiu/T-ZVD ==
  ref : Inport
  Gain : Gain  Gain=0.25
  Gain1 : Gain  Gain=0.5
  Gain2 : Gain  Gain=0.25
  Sum : Sum  Inputs=+++
  Transport Delay : TransportDelay  DelayTime=0.5
  Transport Delay1 : TransportDelay  DelayTime=0.5
  ref_AZ : Outport
  wires:
  Gain1/1 -> Transport Delay/1
  Gain/1 -> Sum/1
  Transport Delay/1 -> Sum/2
  Sum/1 -> ref_AZ/1
  ref/1 -> Gain/1, Gain2/1, Gain1/1
  Gain2/1 -> Transport Delay1/1
  Transport Delay1/1 -> Sum/3

== system Model_3_Hieu_1_12/Heiu/T-ZVD1 ==
  ref : Inport
  Gain : Gain  Gain=0.25
  Gain1 : Gain  Gain=0.5
  Gain2 : Gain  Gain=0.25
  Sum : Sum  Inputs=+++
  Transport Delay : TransportDelay  DelayTime=particle(i).Position(1,1)
  Transport Delay1 : TransportDelay  DelayTime=particle(i).Position(1,2)
  ref_AZ : Outport
  wires:
  Gain1/1 -> Transport Delay/1
  Gain/1 -> Sum/1
  Transport Delay/1 -> Sum/2
  Sum/1 -> ref_AZ/1
  ref/1 -> Gain/1, Gain2/1, Gain1/1
  Gain2/1 -> Transport Delay1/1
  Transport Delay1/1 -> Sum/3

== system Model_3_Hieu_1_12/Model 3/ADRC 10 ==
  ref : Inport
  x : Inport  Port=2
  Gain : Gain  Gain=Kp
  Gain1 : Gain  Gain=Kd
  Gain2 : Gain  Gain=1/b0
  Observer : Subsystem
  Sum : Sum  Inputs=|+-
  Sum3 : Sum  Inputs=|+-
  Sum4 : Sum  Inputs=|+-
  u : Outport
  wires:
  Sum4/1 -> Gain2/1
  Sum/1 -> Gain/1
  Gain2/1 -> u/1, Observer/1(u)
  x/1 -> Observer/2(x)
  Sum3/1 -> Sum4/1
  Observer/2(x2) -> Gain1/1
  Gain1/1 -> Sum3/2
  Gain/1 -> Sum3/1
  ref/1 -> Sum/1
  Observer/1(x3) -> Sum4/2
  Observer/3(x1) -> Sum/2

== system Model_3_Hieu_1_12/Model 3/ADRC 11 ==
  ref : Inport
  x : Inport  Port=2
  Gain : Gain  Gain=Kp1
  Gain1 : Gain  Gain=Kd1
  Gain2 : Gain  Gain=1/b1
  Observer : Subsystem
  Sum : Sum  Inputs=|+-
  Sum3 : Sum  Inputs=|+-
  Sum4 : Sum  Inputs=|+-
  u : Outport
  wires:
  Sum4/1 -> Gain2/1
  Sum/1 -> Gain/1
  Gain2/1 -> u/1, Observer/1(u)
  x/1 -> Observer/2(x)
  Sum3/1 -> Sum4/1
  Observer/2(x2) -> Gain1/1
  Gain1/1 -> Sum3/2
  Gain/1 -> Sum3/1
  ref/1 -> Sum/1
  Observer/1(x3) -> Sum4/2
  Observer/3(x1) -> Sum/2

== system Model_3_Hieu_1_12/Model 3/ADRC 6 ==
  ref : Inport
  x : Inport  Port=2
  Gain : Gain  Gain=Kp
  Gain1 : Gain  Gain=Kd
  Gain2 : Gain  Gain=1/b0
  Observer : Subsystem
  Sum : Sum  Inputs=|+-
  Sum3 : Sum  Inputs=|+-
  Sum4 : Sum  Inputs=|+-
  u : Outport
  wires:
  Sum4/1 -> Gain2/1
  Sum/1 -> Gain/1
  Gain2/1 -> u/1, Observer/1(u)
  x/1 -> Observer/2(x)
  Sum3/1 -> Sum4/1
  Observer/2(x2) -> Gain1/1
  Gain1/1 -> Sum3/2
  Gain/1 -> Sum3/1
  ref/1 -> Sum/1
  Observer/1(x3) -> Sum4/2
  Observer/3(x1) -> Sum/2

== system Model_3_Hieu_1_12/Model 3/ADRC 7 ==
  ref : Inport
  x : Inport  Port=2
  Gain : Gain  Gain=Kp1
  Gain1 : Gain  Gain=Kd1
  Gain2 : Gain  Gain=1/b1
  Observer : Subsystem
  Sum : Sum  Inputs=|+-
  Sum3 : Sum  Inputs=|+-
  Sum4 : Sum  Inputs=|+-
  u : Outport
  wires:
  Sum4/1 -> Gain2/1
  Sum/1 -> Gain/1
  Gain2/1 -> u/1, Observer/1(u)
  x/1 -> Observer/2(x)
  Sum3/1 -> Sum4/1
  Observer/2(x2) -> Gain1/1
  Gain1/1 -> Sum3/2
  Gain/1 -> Sum3/1
  ref/1 -> Sum/1
  Observer/1(x3) -> Sum4/2
  Observer/3(x1) -> Sum/2

== system Model_3_Hieu_1_12/Model 3/ETM2 ==
  ref_ETm4 : Inport
  ETM1 : Subsystem
  ETM4 : Subsystem
  ref1 : Scope
  ref2 : Scope
  ref3 : Scope
  ref_ETM4 : Outport
  wires:
  ETM1/1(Out1) -> ref2/1, ETM4/1(In1)  "ref_ZV"
  ETM4/1(Out1) -> ref3/1, ref_ETM4/1  "ref_ZV"
  ref_ETm4/1 -> ref1/1, ETM1/1(In1)

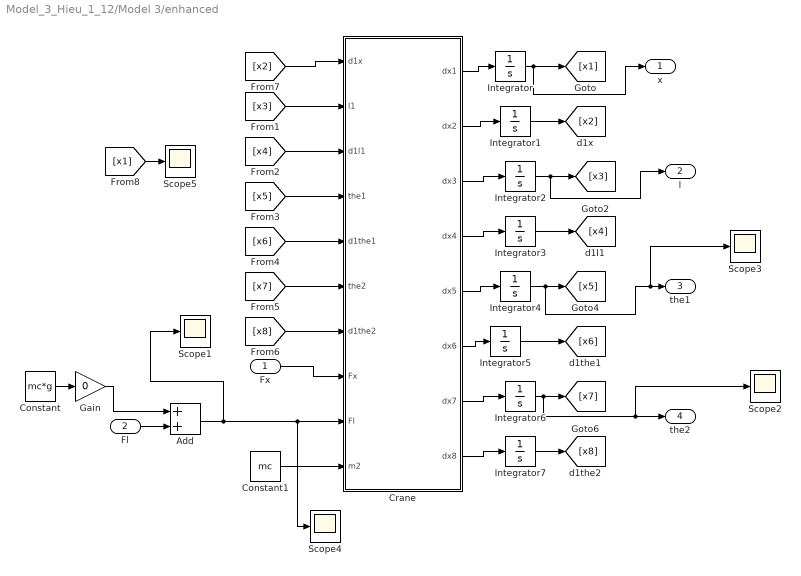
== system Model_3_Hieu_1_12/Model 3/enhanced ==
  Fx : Inport
  Fl : Inport  Port=2
  Add : Sum
  Constant : Constant  Value=mc*g
  Constant1 : Constant  Value=mc
  Crane : MATLAB Function  TreatAsAtomicUnit=on
  Gain : Gain  Gain=0
  Integrator{,1,3,5..7} (6 alike) : Integrator
  Integrator2 : Integrator  InitialCondition=l
  Integrator4 : Integrator  InitialCondition=10*pi/180
  Scope{1..5} (5 alike) : Scope
  x : Outport
  l : Outport  Port=2
  the1 : Outport  Port=3
  the2 : Outport  Port=4
  wires:
  Integrator5/1 -> [x6]
  Integrator2/1 -> l/1, [x3]
  Integrator1/1 -> [x2]
  Integrator/1 -> x/1, [x1]
  Integrator3/1 -> [x4]
  Constant/1 -> Gain/1
  Add/1 -> Scope4/1, Crane/9(Fl), Scope1/1
  Integrator6/1 -> Scope2/1, the2/1, [x7]
  Integrator7/1 -> [x8]
  Crane/1(dx1) -> Integrator/1
  Crane/2(dx2) -> Integrator1/1
  Crane/3(dx3) -> Integrator2/1
  Crane/4(dx4) -> Integrator3/1
  Crane/5(dx5) -> Integrator4/1
  Crane/6(dx6) -> Integrator5/1
  Crane/7(dx7) -> Integrator6/1
  Crane/8(dx8) -> Integrator7/1
  Fx/1 -> Crane/8(Fx)
  Constant1/1 -> Crane/10(m2)
  [x2] -> Crane/1(d1x)
  [x3] -> Crane/2(l1)
  [x4] -> Crane/3(d1l1)
  [x5] -> Crane/4(the1)
  [x6] -> Crane/5(d1the1)
  [x7] -> Crane/6(the2)
  [x8] -> Crane/7(d1the2)
  Integrator4/1 -> Scope3/1, the1/1, [x5]
  Fl/1 -> Add/2
  [x1] -> Scope5/1
  Gain/1 -> Add/1

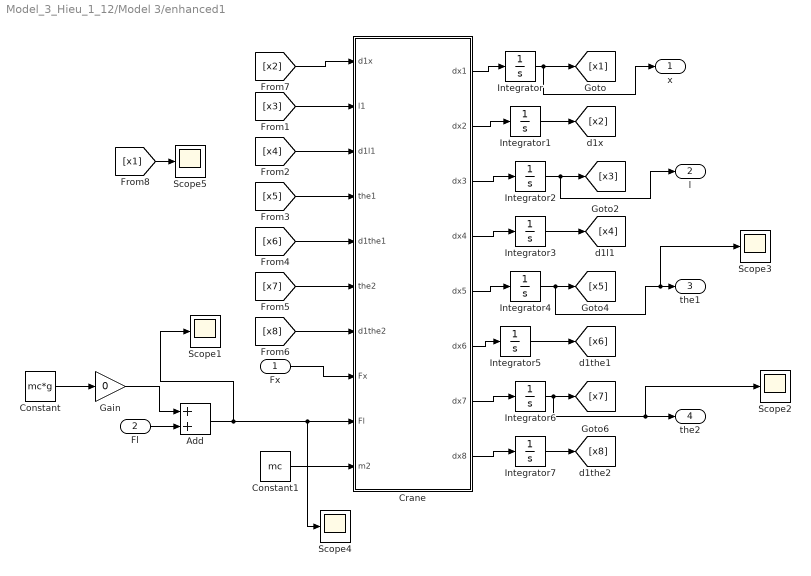
== system Model_3_Hieu_1_12/Model 3/enhanced1 ==
  Fx : Inport
  Fl : Inport  Port=2
  Add : Sum
  Constant : Constant  Value=mc*g
  Constant1 : Constant  Value=mc
  Crane : MATLAB Function  TreatAsAtomicUnit=on
  Gain : Gain  Gain=0
  Integrator{,1,3,5..7} (6 alike) : Integrator
  Integrator2 : Integrator  InitialCondition=l
  Integrator4 : Integrator  InitialCondition=10*pi/180
  Scope{1..5} (5 alike) : Scope
  x : Outport
  l : Outport  Port=2
  the1 : Outport  Port=3
  the2 : Outport  Port=4
  wires:
  Integrator5/1 -> [x6]
  Integrator2/1 -> l/1, [x3]
  Integrator1/1 -> [x2]
  Integrator/1 -> x/1, [x1]
  Integrator3/1 -> [x4]
  Constant/1 -> Gain/1
  Add/1 -> Scope4/1, Crane/9(Fl), Scope1/1
  Integrator6/1 -> Scope2/1, the2/1, [x7]
  Integrator7/1 -> [x8]
  Crane/1(dx1) -> Integrator/1
  Crane/2(dx2) -> Integrator1/1
  Crane/3(dx3) -> Integrator2/1
  Crane/4(dx4) -> Integrator3/1
  Crane/5(dx5) -> Integrator4/1
  Crane/6(dx6) -> Integrator5/1
  Crane/7(dx7) -> Integrator6/1
  Crane/8(dx8) -> Integrator7/1
  Fx/1 -> Crane/8(Fx)
  Constant1/1 -> Crane/10(m2)
  [x2] -> Crane/1(d1x)
  [x3] -> Crane/2(l1)
  [x4] -> Crane/3(d1l1)
  [x5] -> Crane/4(the1)
  [x6] -> Crane/5(d1the1)
  [x7] -> Crane/6(the2)
  [x8] -> Crane/7(d1the2)
  Integrator4/1 -> Scope3/1, the1/1, [x5]
  Fl/1 -> Add/2
  [x1] -> Scope5/1
  Gain/1 -> Add/1

== system Model_3_Hieu_1_12/test_RBF1_2 PSO/ADRC 1 ==
  ref : Inport
  x : Inport  Port=2
  Gain : Gain  Gain=Kp
  Gain1 : Gain  Gain=Kd
  Gain2 : Gain  Gain=1/b0
  Observer : Subsystem
  Sum : Sum  Inputs=|+-
  Sum3 : Sum  Inputs=|+-
  Sum4 : Sum  Inputs=|+-
  u : Outport
  wires:
  Sum4/1 -> Gain2/1
  Sum/1 -> Gain/1
  Gain2/1 -> u/1, Observer/1(u)
  x/1 -> Observer/2(x)
  Sum3/1 -> Sum4/1
  Observer/2(x2) -> Gain1/1
  Gain1/1 -> Sum3/2
  Gain/1 -> Sum3/1
  ref/1 -> Sum/1
  Observer/1(x3) -> Sum4/2
  Observer/3(x1) -> Sum/2

== system Model_3_Hieu_1_12/test_RBF1_2 PSO/ADRC 10 ==
  ref : Inport
  x : Inport  Port=2
  Gain : Gain  Gain=Kp
  Gain1 : Gain  Gain=Kd
  Gain2 : Gain  Gain=1/b0
  Observer : Subsystem
  Sum : Sum  Inputs=|+-
  Sum3 : Sum  Inputs=|+-
  Sum4 : Sum  Inputs=|+-
  u : Outport
  wires:
  Sum4/1 -> Gain2/1
  Sum/1 -> Gain/1
  Gain2/1 -> u/1, Observer/1(u)
  x/1 -> Observer/2(x)
  Sum3/1 -> Sum4/1
  Observer/2(x2) -> Gain1/1
  Gain1/1 -> Sum3/2
  Gain/1 -> Sum3/1
  ref/1 -> Sum/1
  Observer/1(x3) -> Sum4/2
  Observer/3(x1) -> Sum/2

== system Model_3_Hieu_1_12/test_RBF1_2 PSO/ADRC 11 ==
  ref : Inport
  x : Inport  Port=2
  Gain : Gain  Gain=Kp1
  Gain1 : Gain  Gain=Kd1
  Gain2 : Gain  Gain=1/b1
  Observer : Subsystem
  Sum : Sum  Inputs=|+-
  Sum3 : Sum  Inputs=|+-
  Sum4 : Sum  Inputs=|+-
  u : Outport
  wires:
  Sum4/1 -> Gain2/1
  Sum/1 -> Gain/1
  Gain2/1 -> u/1, Observer/1(u)
  x/1 -> Observer/2(x)
  Sum3/1 -> Sum4/1
  Observer/2(x2) -> Gain1/1
  Gain1/1 -> Sum3/2
  Gain/1 -> Sum3/1
  ref/1 -> Sum/1
  Observer/1(x3) -> Sum4/2
  Observer/3(x1) -> Sum/2

== system Model_3_Hieu_1_12/test_RBF1_2 PSO/ADRC 2 ==
  ref : Inport
  x : Inport  Port=2
  Gain : Gain  Gain=Kp1
  Gain1 : Gain  Gain=Kd1
  Gain2 : Gain  Gain=1/b1
  Observer : Subsystem
  Sum : Sum  Inputs=|+-
  Sum3 : Sum  Inputs=|+-
  Sum4 : Sum  Inputs=|+-
  u : Outport
  wires:
  Sum4/1 -> Gain2/1
  Sum/1 -> Gain/1
  Gain2/1 -> u/1, Observer/1(u)
  x/1 -> Observer/2(x)
  Sum3/1 -> Sum4/1
  Observer/2(x2) -> Gain1/1
  Gain1/1 -> Sum3/2
  Gain/1 -> Sum3/1
  ref/1 -> Sum/1
  Observer/1(x3) -> Sum4/2
  Observer/3(x1) -> Sum/2

== system Model_3_Hieu_1_12/test_RBF1_2 PSO/ADRC 3 ==
  ref : Inport
  x : Inport  Port=2
  Gain : Gain  Gain=Kp
  Gain1 : Gain  Gain=Kd
  Gain2 : Gain  Gain=1/b0
  Observer : Subsystem
  Sum : Sum  Inputs=|+-
  Sum3 : Sum  Inputs=|+-
  Sum4 : Sum  Inputs=|+-
  u : Outport
  wires:
  Sum4/1 -> Gain2/1
  Sum/1 -> Gain/1
  Gain2/1 -> u/1, Observer/1(u)
  x/1 -> Observer/2(x)
  Sum3/1 -> Sum4/1
  Observer/2(x2) -> Gain1/1
  Gain1/1 -> Sum3/2
  Gain/1 -> Sum3/1
  ref/1 -> Sum/1
  Observer/1(x3) -> Sum4/2
  Observer/3(x1) -> Sum/2

== system Model_3_Hieu_1_12/test_RBF1_2 PSO/ADRC 4 ==
  ref : Inport
  x : Inport  Port=2
  Gain : Gain  Gain=Kp1
  Gain1 : Gain  Gain=Kd1
  Gain2 : Gain  Gain=1/b1
  Observer : Subsystem
  Sum : Sum  Inputs=|+-
  Sum3 : Sum  Inputs=|+-
  Sum4 : Sum  Inputs=|+-
  u : Outport
  wires:
  Sum4/1 -> Gain2/1
  Sum/1 -> Gain/1
  Gain2/1 -> u/1, Observer/1(u)
  x/1 -> Observer/2(x)
  Sum3/1 -> Sum4/1
  Observer/2(x2) -> Gain1/1
  Gain1/1 -> Sum3/2
  Gain/1 -> Sum3/1
  ref/1 -> Sum/1
  Observer/1(x3) -> Sum4/2
  Observer/3(x1) -> Sum/2

== system Model_3_Hieu_1_12/test_RBF1_2 PSO/ADRC 5 ==
  ref : Inport
  x : Inport  Port=2
  Gain : Gain  Gain=Kp
  Gain1 : Gain  Gain=Kd
  Gain2 : Gain  Gain=1/b0
  Observer : Subsystem
  Sum : Sum  Inputs=|+-
  Sum3 : Sum  Inputs=|+-
  Sum4 : Sum  Inputs=|+-
  u : Outport
  wires:
  Sum4/1 -> Gain2/1
  Sum/1 -> Gain/1
  Gain2/1 -> u/1, Observer/1(u)
  x/1 -> Observer/2(x)
  Sum3/1 -> Sum4/1
  Observer/2(x2) -> Gain1/1
  Gain1/1 -> Sum3/2
  Gain/1 -> Sum3/1
  ref/1 -> Sum/1
  Observer/1(x3) -> Sum4/2
  Observer/3(x1) -> Sum/2

== system Model_3_Hieu_1_12/test_RBF1_2 PSO/ADRC 6 ==
  ref : Inport
  x : Inport  Port=2
  Gain : Gain  Gain=Kp1
  Gain1 : Gain  Gain=Kd1
  Gain2 : Gain  Gain=1/b1
  Observer : Subsystem
  Sum : Sum  Inputs=|+-
  Sum3 : Sum  Inputs=|+-
  Sum4 : Sum  Inputs=|+-
  u : Outport
  wires:
  Sum4/1 -> Gain2/1
  Sum/1 -> Gain/1
  Gain2/1 -> u/1, Observer/1(u)
  x/1 -> Observer/2(x)
  Sum3/1 -> Sum4/1
  Observer/2(x2) -> Gain1/1
  Gain1/1 -> Sum3/2
  Gain/1 -> Sum3/1
  ref/1 -> Sum/1
  Observer/1(x3) -> Sum4/2
  Observer/3(x1) -> Sum/2

== system Model_3_Hieu_1_12/test_RBF1_2 PSO/ETM2 ==
  ref_ETm4 : Inport
  ETM1 : Subsystem
  ETM4 : Subsystem
  ref1 : Scope
  ref2 : Scope
  ref3 : Scope
  ref_ETM4 : Outport
  wires:
  ETM1/1(Out1) -> ref2/1, ETM4/1(In1)  "ref_ZV"
  ETM4/1(Out1) -> ref3/1, ref_ETM4/1  "ref_ZV"
  ref_ETm4/1 -> ref1/1, ETM1/1(In1)

== system Model_3_Hieu_1_12/test_RBF1_2 PSO/ETM4 ==
  In1 : Inport
  Gain : Gain  Gain=A1_etm4_2
  Gain1 : Gain  Gain=A2_etm4_2
  Gain2 : Gain  Gain=A3_etm4_2
  Gain3 : Gain  Gain=A4_etm4_2
  Sum : Sum  Inputs=++++
  Transport Delay : TransportDelay  DelayTime=t1_etm4_2
  Transport Delay1 : TransportDelay  DelayTime=t2_etm4_2
  Transport Delay2 : TransportDelay  DelayTime=t3_etm4_2
  ref : Outport
  wires:
  In1/1 -> Gain1/1, Gain3/1, Gain2/1, Gain/1
  Gain1/1 -> Transport Delay/1
  Transport Delay/1 -> Sum/2
  Sum/1 -> ref/1
  Gain2/1 -> Transport Delay1/1
  Gain/1 -> Sum/1
  Transport Delay1/1 -> Sum/3
  Gain3/1 -> Transport Delay2/1
  Transport Delay2/1 -> Sum/4

== system Model_3_Hieu_1_12/test_RBF1_2 PSO/Fitness APS 1 ==
  e : Inport
  Abs : Abs
  Abs1 : Abs
  Integrator : Integrator
  MinMax Running Resettable : simulink/Math Operations/MinMax Running Resettable  Function=max  vinit=0.0
  Step : Step  Time=0.000001  Before=1  After=0  SampleTime=0
  IAE : Outport
  MAx : Outport  Port=2
  wires:
  Abs/1 -> Integrator/1
  Abs1/1 -> MinMax Running Resettable/1
  Step/1 -> MinMax Running Resettable/2
  e/1 -> Abs/1, Abs1/1
  Integrator/1 -> IAE/1
  MinMax Running Resettable/1 -> MAx/1

== system Model_3_Hieu_1_12/test_RBF1_2 PSO/Fitness APS 2 ==
  e : Inport
  Abs : Abs
  Abs1 : Abs
  Integrator : Integrator
  MinMax Running Resettable : simulink/Math Operations/MinMax Running Resettable  Function=max  vinit=0.0
  Step : Step  Time=0.000001  Before=1  After=0  SampleTime=0
  IAE : Outport
  MAx : Outport  Port=2
  wires:
  Abs/1 -> Integrator/1
  Abs1/1 -> MinMax Running Resettable/1
  Step/1 -> MinMax Running Resettable/2
  e/1 -> Abs/1, Abs1/1
  Integrator/1 -> IAE/1
  MinMax Running Resettable/1 -> MAx/1

== system Model_3_Hieu_1_12/test_RBF1_2 PSO/PSO-ETM1 ==
  In1 : Inport
  Input : Inport  Port=2
  Input1 : Inport  Port=3
  Input2 : Inport  Port=4
  Gain : Gain  Gain=0.1667
  Gain1 : Gain  Gain=0.3333
  Gain2 : Gain  Gain=0.3333
  Gain3 : Gain  Gain=0.1667
  Sum : Sum  Inputs=++++
  Variable Transport Delay : VariableTransportDelay  VariableDelayType=Variable transport delay  MaximumDelay=10
  Variable Transport Delay1 : VariableTransportDelay  VariableDelayType=Variable transport delay  MaximumDelay=10
  Variable Transport Delay2 : VariableTransportDelay  VariableDelayType=Variable transport delay  MaximumDelay=10
  Out1 : Outport
  wires:
  In1/1 -> Gain1/1, Gain3/1, Gain2/1, Gain/1
  Gain1/1 -> Variable Transport Delay/1
  Variable Transport Delay/1 -> Sum/2
  Sum/1 -> Out1/1
  Gain2/1 -> Variable Transport Delay1/1
  Gain/1 -> Sum/1
  Variable Transport Delay1/1 -> Sum/3
  Gain3/1 -> Variable Transport Delay2/1
  Variable Transport Delay2/1 -> Sum/4
  Input/1 -> Variable Transport Delay/2
  Input1/1 -> Variable Transport Delay1/2
  Input2/1 -> Variable Transport Delay2/2

== system Model_3_Hieu_1_12/test_RBF1_2 PSO/PSO-ETM2 ==
  In1 : Inport
  Input : Inport  Port=2
  Input1 : Inport  Port=3
  Input2 : Inport  Port=4
  Gain : Gain  Gain=0.1667
  Gain1 : Gain  Gain=0.3333
  Gain2 : Gain  Gain=0.3333
  Gain3 : Gain  Gain=0.1667
  Sum : Sum  Inputs=++++
  Variable Transport Delay : VariableTransportDelay  VariableDelayType=Variable transport delay  MaximumDelay=10
  Variable Transport Delay1 : VariableTransportDelay  VariableDelayType=Variable transport delay  MaximumDelay=10
  Variable Transport Delay2 : VariableTransportDelay  VariableDelayType=Variable transport delay  MaximumDelay=10
  ref : Outport
  wires:
  In1/1 -> Gain1/1, Gain3/1, Gain2/1, Gain/1
  Gain1/1 -> Variable Transport Delay/1
  Variable Transport Delay/1 -> Sum/2
  Sum/1 -> ref/1
  Gain2/1 -> Variable Transport Delay1/1
  Gain/1 -> Sum/1
  Variable Transport Delay1/1 -> Sum/3
  Gain3/1 -> Variable Transport Delay2/1
  Variable Transport Delay2/1 -> Sum/4
  Input/1 -> Variable Transport Delay/2
  Input1/1 -> Variable Transport Delay1/2
  Input2/1 -> Variable Transport Delay2/2

== system Model_3_Hieu_1_12/test_RBF1_2 PSO/PSO-ETM4 ==
  In1 : Inport
  Input : Inport  Port=2
  Input1 : Inport  Port=3
  Input2 : Inport  Port=4
  Gain : Gain  Gain=0.1667
  Gain1 : Gain  Gain=0.3333
  Gain2 : Gain  Gain=0.3333
  Gain3 : Gain  Gain=0.1667
  Sum : Sum  Inputs=++++
  Variable Transport Delay : VariableTransportDelay  VariableDelayType=Variable transport delay  MaximumDelay=10
  Variable Transport Delay1 : VariableTransportDelay  VariableDelayType=Variable transport delay  MaximumDelay=10
  Variable Transport Delay2 : VariableTransportDelay  VariableDelayType=Variable transport delay  MaximumDelay=10
  Out1 : Outport
  wires:
  In1/1 -> Gain1/1, Gain3/1, Gain2/1, Gain/1
  Gain1/1 -> Variable Transport Delay/1
  Variable Transport Delay/1 -> Sum/2
  Sum/1 -> Out1/1
  Gain2/1 -> Variable Transport Delay1/1
  Gain/1 -> Sum/1
  Variable Transport Delay1/1 -> Sum/3
  Gain3/1 -> Variable Transport Delay2/1
  Variable Transport Delay2/1 -> Sum/4
  Input/1 -> Variable Transport Delay/2
  Input1/1 -> Variable Transport Delay1/2
  Input2/1 -> Variable Transport Delay2/2
